simulink model "part4a"  (R2018a)
settings: Solver=VariableStepAuto  StartTime=0.0  StopTime=4000  RelTol=1e-3
values from neighbouring files (symbols this model uses):
  ain = 90    [variables.m]
  c = 16    [variables.m]
  qin = 10*.134/60    (= 0.0223333333333)    [variables.m]
settings Model: Creator=jschm  LastModifiedBy=jschm

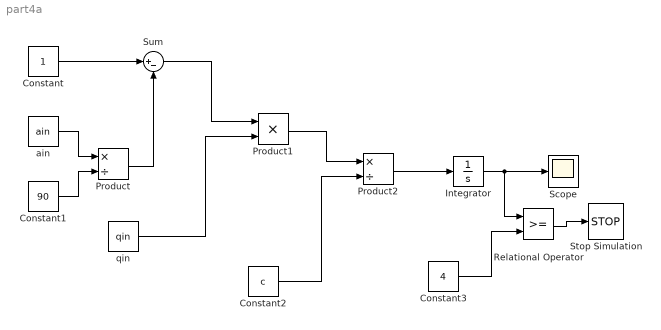
== system part4a ==
  Constant : Constant
  Constant1 : Constant  Value=90
  Constant2 : Constant  Value=c
  Constant3 : Constant  Value=4
  Integrator : Integrator
  Product : Product  Inputs=*/
  Product1 : Product
  Product2 : Product  Inputs=*/
  Relational Operator : RelationalOperator  OutDataTypeStr=boolean  RndMeth=Simplest
  Scope : Scope
  Stop Simulation : Stop
  Sum : Sum  Inputs=|+-
  ain : Constant  Value=ain
  "qin " : Constant  Value=qin
  wires:
  Constant/1 -> Sum/1
  Constant1/1 -> Product/2
  ain/1 -> Product/1
  Product/1 -> Sum/2
  Sum/1 -> Product1/1
  "qin "/1 -> Product1/2
  Product1/1 -> Product2/1
  Constant2/1 -> Product2/2
  Product2/1 -> Integrator/1
  Integrator/1 -> Relational Operator/1, Scope/1
  Relational Operator/1 -> Stop Simulation/1
  Constant3/1 -> Relational Operator/2
